simulink model "simulink_pd"  (Simulink 8.5)
settings: Solver=ode45  StartTime=0.0  StopTime=100  FixedStep=0.05  RelTol=1e-3
settings Model: Creator=SuseongKim  LastModifiedBy=LSI
settings DebuggingCC: SolverPrmCheckMsg=warning  FcnCallInpInsideContextMsg=UseLocalSettings

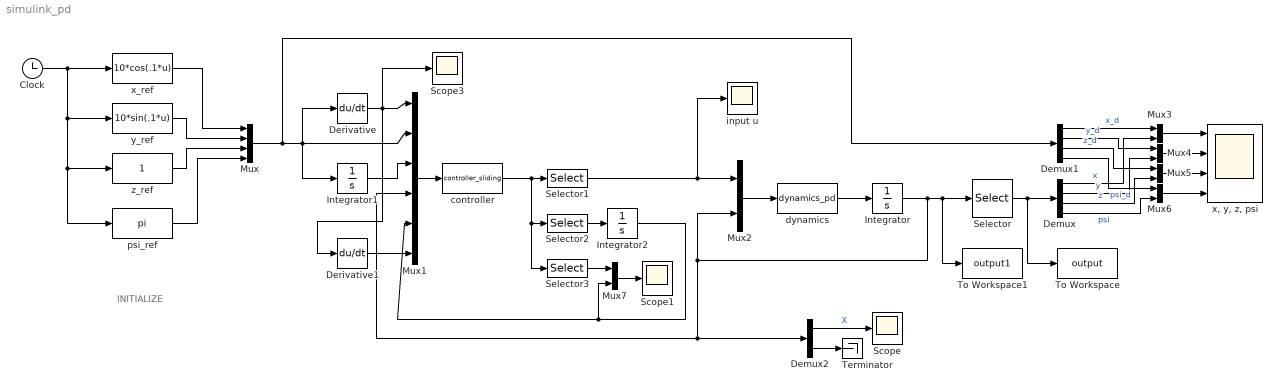
== system simulink_pd ==
  note: INITIALIZE
  Clock : Clock
  Demux : Demux
  Demux1 : Demux
  Demux2 : Demux  Outputs=2
  Derivative : Derivative
  Derivative1 : Derivative
  Integrator : Integrator  InitialCondition=[0 0 0 0 0 0 0 0 0 0 0 0]
  Integrator1 : Integrator  InitialCondition=[0 0 0 0]
  Integrator2 : Integrator  InitialCondition=[0 0]
  Mux : Mux
  Mux1 : Mux  Inputs=6
  Mux{2..7} (6 alike) : Mux  Inputs=2
  Scope : Scope
  Scope1 : Scope
      settings: SaveName=ScopeData4
  Scope3 : Scope
      settings: SaveName=ScopeData3
  Selector : Selector  InputPortWidth=12  Indices=[1 2 3 6]
  Selector1 : Selector  InputPortWidth=8  Indices=[1 2 3 4]
  Selector2 : Selector  InputPortWidth=8  Indices=[7 8]
  Selector3 : Selector  InputPortWidth=8  Indices=[5 6]
  Terminator : Terminator
  To Workspace : ToWorkspace  VariableName=output  SampleTime=-1
  To Workspace1 : ToWorkspace  VariableName=output1  SampleTime=-1
  controller : MATLABFcn  MATLABFcn=controller_sliding  OutputDimensions=8
  dynamics : MATLABFcn  MATLABFcn=dynamics_pd  OutputDimensions=12
  input u : Scope
      settings: ShowLegends=on  TimeRange=30  YMin=-50  YMax=350  SaveName=ScopeData2
  psi_ref : Fcn  Expr=pi
  "x, y, z, psi" : Scope  NumInputPorts=4
      settings: ShowLegends=on  TimeRange=0.2425876010781671  YMin=0~0~0~0  YMax=10~0.25~0.05~3.5
  x_ref : Fcn  Expr=10*cos(.1*u)
  y_ref : Fcn  Expr=10*sin(.1*u)
  z_ref : Fcn  Expr=1
  wires:
  Mux/1 -> Integrator1/1, Mux1/2, Derivative/1, Demux1/1
  dynamics/1 -> Integrator/1
  Integrator/1 -> Mux1/4, Demux2/1, Mux2/2, To Workspace1/1, Selector/1
  Mux1/1 -> controller/1
  Mux2/1 -> dynamics/1
  controller/1 -> Selector3/1, Selector2/1, Selector1/1
  Derivative/1 -> Derivative1/1, Scope3/1, Mux1/1
  Demux/1 -> Mux3/2  "x"
  Demux/2 -> Mux4/2  "y"
  Demux/3 -> Mux5/2  "z"
  Demux/4 -> Mux6/2  "psi"
  Selector/1 -> Demux/1, To Workspace/1
  Demux1/1 -> Mux3/1  "x_d"
  Demux1/2 -> Mux4/1  "y_d"
  Demux1/3 -> Mux5/1  "z_d"
  Demux1/4 -> Mux6/1  "psi_d"
  y_ref/1 -> Mux/2
  psi_ref/1 -> Mux/4
  z_ref/1 -> Mux/3
  x_ref/1 -> Mux/1
  Clock/1 -> y_ref/1, psi_ref/1, z_ref/1, x_ref/1
  Integrator1/1 -> Mux1/3
  Mux3/1 -> "x, y, z, psi"/1
  Mux4/1 -> "x, y, z, psi"/2
  Mux5/1 -> "x, y, z, psi"/3
  Mux6/1 -> "x, y, z, psi"/4
  Demux2/1 -> Scope/1  "X"
  Demux2/2 -> Terminator/1
  Selector1/1 -> input u/1, Mux2/1
  Selector2/1 -> Integrator2/1
  Integrator2/1 -> Mux7/2, Mux1/5
  Mux7/1 -> Scope1/1
  Selector3/1 -> Mux7/1
  Derivative1/1 -> Mux1/6
